simulink model "P3simulink2022a"  (R2022a)
settings: Solver=VariableStepAuto  StartTime=0.0  StopTime=10.0  RelTol=1e-3
values from neighbouring files (symbols this model uses):
  K1 = -1    [P3.m]
  K2 = -0.8    [P3.m]
  Treshold_y = 10    [P3.m]
  V = 0    [P1.m]    (also in P2.m = 15; P3.m = 15; P4.m = 15; QuiverTest.m = zeros(length(U),length(U)) -g)
  Vy_Inicial = 1    [P3.m]
libraries: simulink x2
settings Model: Creator=TERESA NOGUEIRA  LastModifiedBy=TERESA NOGUEIRA
settings SolverCC: ZeroCrossAlgorithm=Adaptive
settings ModelReferenceCC: EnableRefExpFcnMdlSchedulingChecks=off
settings RTWCC: Description=Generic Real-Time Target

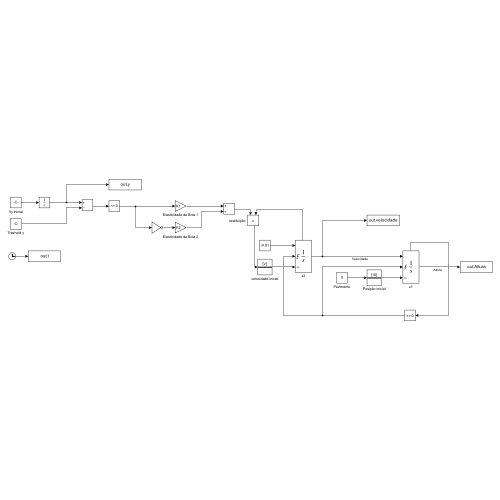
[thumbnail: Simulink's stored preview of the top-level diagram]
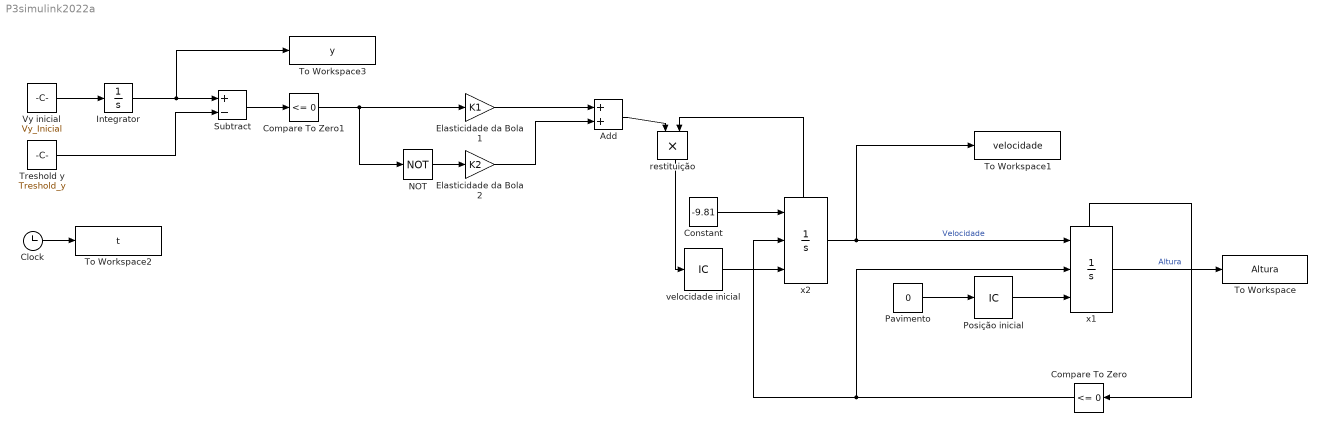
== system P3simulink2022a ==
  Add : Sum
  Clock : Clock
      settings: Decimation=200
  Compare To Zero : simulink/Logic and Bit Operations/Compare To Zero  relop=<=  OutDataTypeStr=boolean
  Compare To Zero1 : simulink/Logic and Bit Operations/Compare To Zero  relop=<=  OutDataTypeStr=boolean
  Constant : Constant  Value=-9.81
  Elasticidade da Bola 1 : Gain  Gain=K1
  Elasticidade da Bola 2 : Gain  Gain=K2
  Integrator : Integrator  ContinuousStateAttributes='xpos'
  NOT : Logic  Operator=NOT  IconShape=distinctive  AllPortsSameDT=off  OutDataTypeStr=boolean
  Pavimento : Constant  Value=0
  Posição inicial : InitialCondition  Value=10
  Subtract : Sum  Inputs=+-
  To Workspace : ToWorkspace  VariableName=Altura  SampleTime=-1
      settings: Save2DSignal=2-D array (concatenate along first dimension)
  To Workspace1 : ToWorkspace  VariableName=velocidade  SampleTime=-1
      settings: Save2DSignal=2-D array (concatenate along first dimension)
  To Workspace2 : ToWorkspace  VariableName=t  SampleTime=-1
      settings: Save2DSignal=2-D array (concatenate along first dimension)
  To Workspace3 : ToWorkspace  VariableName=y  SampleTime=-1
  Treshold y : Constant  Value=Treshold_y
  Vy inicial : Constant  Value=Vy_Inicial
  restituição : Product
  velocidade inicial : InitialCondition  Value=V
  x1 : Integrator  ExternalReset=rising  InitialConditionSource=external  ShowStatePort=on
  x2 : Integrator  ExternalReset=rising  InitialConditionSource=external  ShowStatePort=on
  wires:
  Vy inicial/1 -> Integrator/1
  Integrator/1 -> Subtract/1, To Workspace3/1
  x2/1 -> To Workspace1/1, x1/1  "Velocidade"
  velocidade inicial/1 -> x2/3
  Posição inicial/1 -> x1/3
  Constant/1 -> x2/1
  Clock/1 -> To Workspace2/1
  x1/1 -> To Workspace/1  "Altura"
  x1/State -> Compare To Zero/1
  Compare To Zero/1 -> x2/2, x1/2
  Pavimento/1 -> Posição inicial/1
  Treshold y/1 -> Subtract/2
  Subtract/1 -> Compare To Zero1/1
  Elasticidade da Bola 1/1 -> Add/1
  Elasticidade da Bola 2/1 -> Add/2
  Add/1 -> restituição/1
  x2/State -> restituição/2
  restituição/1 -> velocidade inicial/1
  Compare To Zero1/1 -> NOT/1, Elasticidade da Bola 1/1
  NOT/1 -> Elasticidade da Bola 2/1
